simulink subsystem "motorSubsystem"  (R2024a)
settings: Solver=VariableStepAuto  StartTime=0.0  StopTime=10.0  RelTol=1e-3
settings Model: Creator=janho  LastModifiedBy=janho

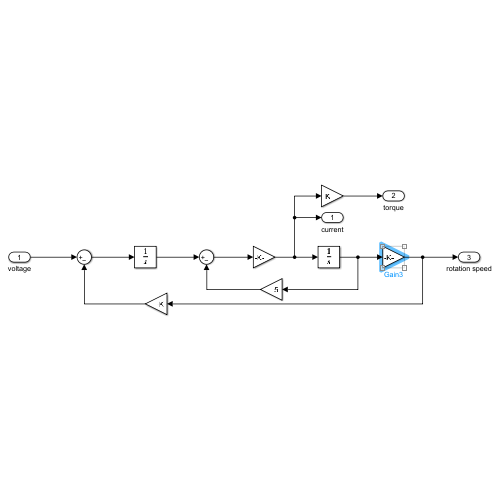
[thumbnail: Simulink's stored preview of the top-level diagram]
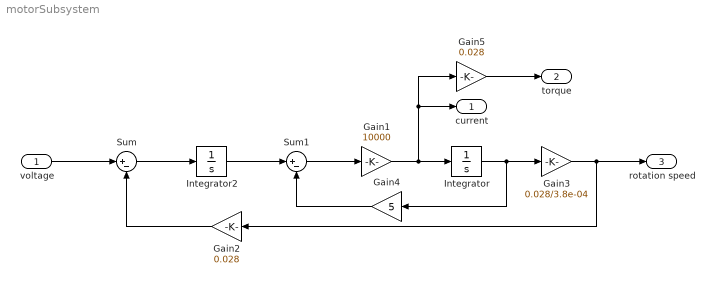
== system motorSubsystem ==
  voltage : Inport
  Gain1 : Gain  Gain=10000
  Gain2 : Gain  Gain=0.028
  Gain3 : Gain  Gain=0.028/3.8e-04
  Gain4 : Gain  Gain=5
  Gain5 : Gain  Gain=0.028
  Integrator : Integrator
  Integrator2 : Integrator
  Sum : Sum  Inputs=|+-
  Sum1 : Sum  Inputs=|+-
  current : Outport
  torque : Outport  Port=2
  rotation speed : Outport  Port=3
  wires:
  Sum/1 -> Integrator2/1
  Integrator/1 -> Gain3/1, Gain4/1
  Gain5/1 -> torque/1
  Sum1/1 -> Gain1/1
  Gain2/1 -> Sum/2
  Gain1/1 -> Integrator/1, current/1, Gain5/1
  Integrator2/1 -> Sum1/1
  Gain4/1 -> Sum1/2
  Gain3/1 -> rotation speed/1, Gain2/1
  voltage/1 -> Sum/1
